simulink model "mt_valid_test"  (R2016b)
settings: Solver=VariableStepAuto  StartTime=0.0  StopTime=10.0  RelTol=1e-3
undefined symbols (not defined in the file): fsw_params, sim_params
libraries: simulink x1, magnetorquer_assembly_lib x1
settings Model: Creator=taylorreynolds  LastModifiedBy=taylorreynolds

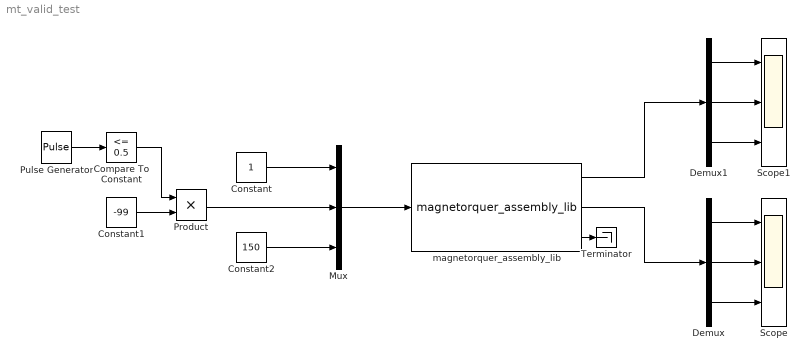
== system mt_valid_test ==
  Compare To Constant : simulink/Logic and Bit Operations/Compare To Constant  relop=<=  const=0.5  OutDataTypeStr=uint8
  Constant : Constant
  Constant1 : Constant  Value=-99
  Constant2 : Constant  Value=150
  Demux : Demux  Outputs=3
  Demux1 : Demux  Outputs=3
  Mux : Mux  Inputs=3
  Product : Product
  Pulse Generator : DiscretePulseGenerator  PulseType=Time based  Period=sim_params.telecom.sync_pulse_s  PulseWidth=fsw_params.actuators.pct_sync_pulse
  Scope : Scope  NumInputPorts=3
  Scope1 : Scope  NumInputPorts=3
  Terminator : Terminator
  magnetorquer_assembly_lib : magnetorquer_assembly_lib/magnetorquer_assembly_lib
  wires:
  Mux/1 -> magnetorquer_assembly_lib/1
  Constant/1 -> Mux/1
  Product/1 -> Mux/2
  Constant2/1 -> Mux/3
  magnetorquer_assembly_lib/2 -> Demux/1
  Demux/2 -> Scope/2
  Demux/1 -> Scope/1
  Demux/3 -> Scope/3
  magnetorquer_assembly_lib/1 -> Demux1/1
  Demux1/2 -> Scope1/2
  Demux1/1 -> Scope1/1
  Demux1/3 -> Scope1/3
  magnetorquer_assembly_lib/3 -> Terminator/1
  Pulse Generator/1 -> Compare To Constant/1
  Constant1/1 -> Product/2
  Compare To Constant/1 -> Product/1
